simulink model "Parm_track_ieee"  (R2021a)
settings: Solver=ode8  StartTime=0.0  StopTime=FB_current.time(end)  FixedStep=ts  RelTol=1e-3
undefined symbols (not defined in the file): As, Bs, c1, c2, Cs, Ds, k, lambda, LipFT, LipI2T, p, p2, qmax, r1, r2, r3, ts, Tse
libraries: simulink x11
settings Model: SimulationMode=accelerator  Creator=Usuario  LastModifiedBy=pedro
settings SolverCC: AlgebraicLoopSolver=TrustRegion
settings DataIOCC: ExternalInput=FBI(i)  LoadExternalInput=on  SaveOutput=off  SignalLogging=off  DSMLogging=off  SaveTime=off  ReturnWorkspaceOutputs=off
settings DebuggingCC: SFMachineParentedDataDiag=warning  ArithmeticOperatorsInVariantConditions=warning
settings SFSimCC: SimUseLocalCustomCode=off  CustomCodeUndefinedFunction=UseInterfaceOnly
settings RTWCC: RTWUseLocalCustomCode=off

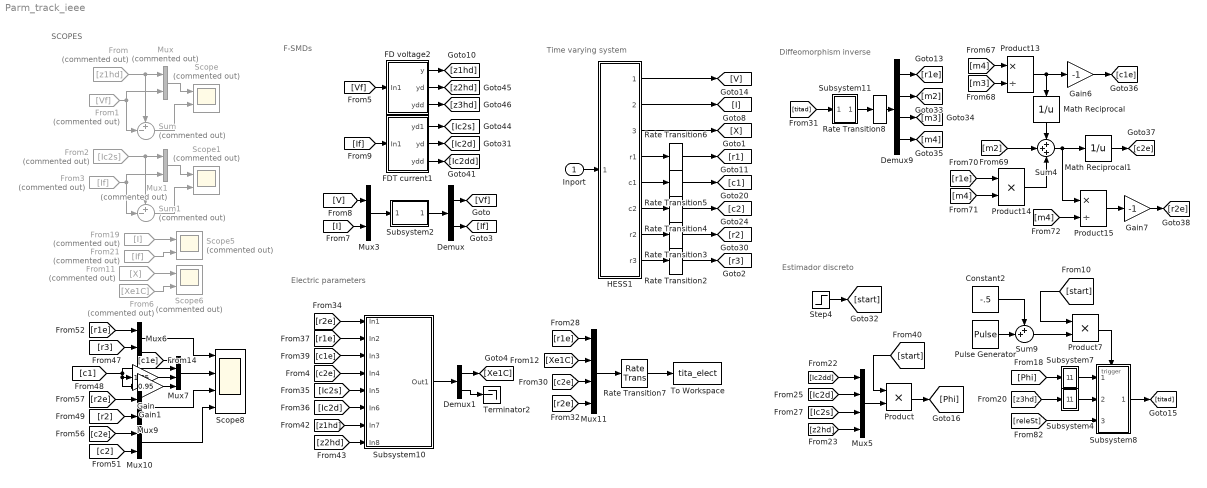
== system Parm_track_ieee ==
  note: Estimador discreto
  note: SCOPES
  note: F-SMDs
  note: Time varying system
  note: Diffeomorphism inverse
  note: Electric parameters
  Inport : Inport
  Constant2 : Constant  Value=-.5
  Demux : Demux  Outputs=2
  Demux1 : Demux  Outputs=2
  Demux9 : Demux
  FD voltage2 : Subsystem
  FDT current1 : Subsystem
  From : From  Commented=on  GotoTag=z1hd
  From1 : From  Commented=on  GotoTag=Vf
  From11 : From  Commented=on  GotoTag=X
  From19 : From  Commented=on  GotoTag=I
  From2 : From  Commented=on  GotoTag=Ic2s
  From21 : From  Commented=on  GotoTag=If
  From3 : From  Commented=on  GotoTag=If
  From6 : From  Commented=on  GotoTag=Xe1C
  Gain : Gain  Gain=1.05
  Gain1 : Gain  Gain=0.95
  Gain6 : Gain  Gain=-1
  Gain7 : Gain  Gain=-1
  HESS1 : Subsystem
  Math Reciprocal : Math  Operator=reciprocal  SignedPower=on  SaturateOnIntegerOverflow=on
  Math Reciprocal1 : Math  Operator=reciprocal  SignedPower=on  SaturateOnIntegerOverflow=on
  Mux : Mux  Commented=on  Inputs=2
  Mux1 : Mux  Commented=on  Inputs=2
  Mux{3,6,9..10} (4 alike) : Mux  Inputs=2
  Mux11 : Mux
  Mux5 : Mux
  Mux7 : Mux
  Product : Product
  Product13 : Product  Inputs=*/
  Product14 : Product
  Product15 : Product  Inputs=*/
  Product7 : Product
  Pulse Generator : DiscretePulseGenerator  PulseType=Time based  Period=Tse  PulseWidth=50
  Rate Transition{2..6,8} (6 alike) : RateTransition  OutPortSampleTime=Tse
  Rate Transition7 : RateTransition  OutPortSampleTime=Tse*2000
  Scope{,1,5..6} (4 alike) : Scope  Commented=on  NumInputPorts=2
  Scope8 : Scope  NumInputPorts=4
  Step4 : Step  Time=30  SampleTime=0
  Subsystem10 : Subsystem
  Subsystem11 : Subsystem
  Subsystem2 : Subsystem
  Subsystem4 : Subsystem
  Subsystem7 : Subsystem
  Subsystem8 : Subsystem
  Sum : Sum  Commented=on  Inputs=+-|
  Sum1 : Sum  Commented=on  Inputs=+-|
  Sum4 : Sum  Inputs=+++
  Sum9 : Sum  Inputs=++|
  Terminator2 : Terminator
  To Workspace : ToWorkspace  VariableName=tita_elect  SaveFormat=Structure With Time  SampleTime=-1
  wires:
  Subsystem2/1(Out1) -> Demux/1
  Demux/1 -> [Vf]
  [V] -> Mux3/1
  Demux/2 -> [If]
  Mux3/1 -> Subsystem2/1(In1)
  HESS1/1(Tensión) -> [V]
  HESS1/2(Corriente) -> [I]
  FD voltage2/2(yd) -> [z2hd]
  FDT current1/1(yd1) -> [Ic2s]
  FD voltage2/1(y) -> [z1hd]
  FDT current1/2(yd) -> [Ic2d]
  [Vf] -> FD voltage2/1(In1)
  FDT current1/3(ydd) -> [Ic2dd]
  [I] -> Mux3/2
  [If] -> FDT current1/1(In1)
  FD voltage2/3(ydd) -> [z3hd]
  Inport/1 -> HESS1/1(Inport)
  HESS1/5(c1) -> Rate Transition5/1
  HESS1/4(r1) -> Rate Transition6/1
  HESS1/6(c2) -> Rate Transition4/1
  HESS1/8(r3) -> Rate Transition2/1
  HESS1/7(r2) -> Rate Transition3/1
  HESS1/3("Estados ") -> [X]
  From/1 -> Mux/1, Sum/1
  From1/1 -> Sum/2, Mux/2
  Mux/1 -> Scope/1
  Sum/1 -> Scope/2
  Sum1/1 -> Scope1/2
  Mux1/1 -> Scope1/1
  From3/1 -> Mux1/2, Sum1/2
  From2/1 -> Sum1/1, Mux1/1
  [releSt] -> Subsystem8/3(In3)
  Subsystem8/1(Output) -> [titad]
  Subsystem4/1(Out1) -> Subsystem8/2(In2)
  Pulse Generator/1 -> Sum9/2
  [Ic2dd] -> Mux5/1
  Mux5/1 -> Product/2
  [z2hd] -> Mux5/4
  Product/1 -> [Phi]
  [z3hd] -> Subsystem4/1(In1)
  Sum9/1 -> Product7/2
  [Ic2s] -> Mux5/3
  Subsystem7/1(Out1) -> Subsystem8/1(In1)
  [Ic2d] -> Mux5/2
  [Phi] -> Subsystem7/1(In1)
  Step4/1 -> [start]
  [m4] -> Product13/1
  [m4] -> Product15/2
  Math Reciprocal/1 -> Sum4/1
  Demux9/3 -> [m3]
  Math Reciprocal1/1 -> [c2e]
  Demux9/1 -> [r1e]
  Demux9/4 -> [m4]
  [m4] -> Product14/2
  [m3] -> Product13/2
  Gain7/1 -> [r2e]
  [r1e] -> Product14/1
  Demux9/2 -> [m2]
  Product15/1 -> Gain7/1
  [m2] -> Sum4/2
  Gain6/1 -> [c1e]
  Mux9/1 -> Scope8/3
  Mux7/1 -> Scope8/2
  Gain/1 -> Mux7/3
  [c2] -> Mux10/2
  [c2e] -> Mux10/1
  [r2e] -> Mux9/1
  [r3] -> Mux6/2
  Gain1/1 -> Mux7/4
  Mux6/1 -> Scope8/1
  [r2] -> Mux9/2
  Mux10/1 -> Scope8/4
  [c1] -> Mux7/2, Gain1/1, Gain/1
  [r1e] -> Mux6/1
  From19/1 -> Scope5/1
  From21/1 -> Scope5/2
  Rate Transition2/1 -> [r3]
  Rate Transition3/1 -> [r2]
  Rate Transition4/1 -> [c2]
  Rate Transition5/1 -> [c1]
  Rate Transition6/1 -> [r1]
  [Xe1C] -> Mux11/2
  [r1e] -> Mux11/1
  [c2e] -> Mux11/3
  [r2e] -> Mux11/4
  Mux11/1 -> Rate Transition7/1
  Rate Transition7/1 -> To Workspace/1
  From11/1 -> Scope6/1
  [c1e] -> Mux7/1
  [titad] -> Subsystem11/1(In1)
  Subsystem11/1(Out1) -> Rate Transition8/1
  Rate Transition8/1 -> Demux9/1
  Product13/1 -> Math Reciprocal/1, Gain6/1
  Product14/1 -> Sum4/3
  Sum4/1 -> Product15/1, Math Reciprocal1/1
  [start] -> Product7/1
  Constant2/1 -> Sum9/1
  [start] -> Product/1
  Product7/1 -> Subsystem8/Trigger
  [z1hd] -> Subsystem10/7(In7)
  Subsystem10/1(Out1) -> Demux1/1
  [Ic2d] -> Subsystem10/6(In6)
  [z2hd] -> Subsystem10/8(In8)
  [Ic2s] -> Subsystem10/5(In5)
  Demux1/2 -> Terminator2/1
  [r1e] -> Subsystem10/2(In2)
  [c2e] -> Subsystem10/4(In4)
  Demux1/1 -> [Xe1C]
  [r2e] -> Subsystem10/1(In1)
  [c1e] -> Subsystem10/3(In3)
  From6/1 -> Scope6/2

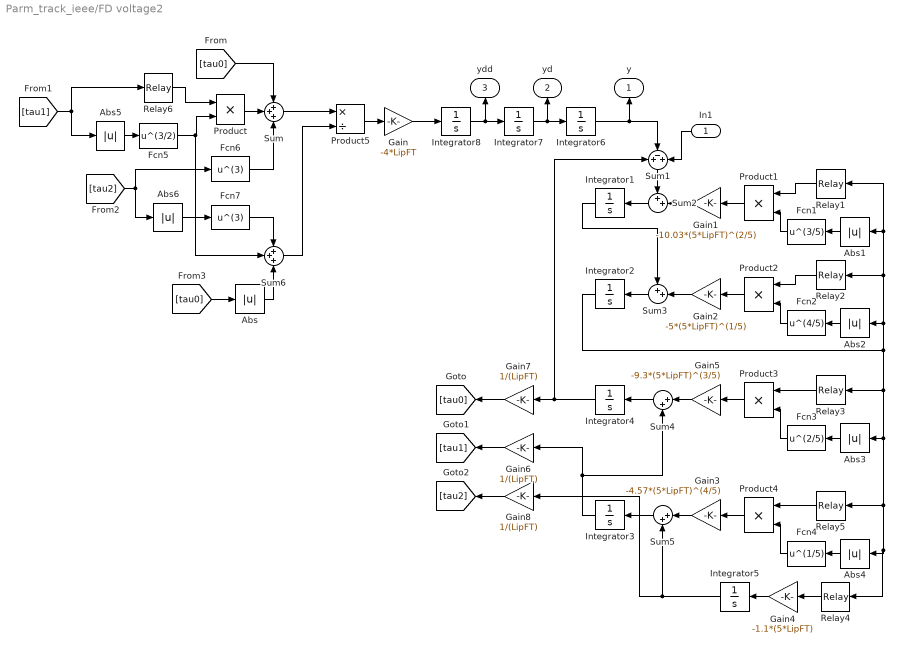
== system Parm_track_ieee/FD voltage2 ==
  In1 : Inport
  Abs{,1..6} (7 alike) : Abs
  Fcn1 : Fcn  Expr=u^(3/5)
  Fcn2 : Fcn  Expr=u^(4/5)
  Fcn3 : Fcn  Expr=u^(2/5)
  Fcn4 : Fcn  Expr=u^(1/5)
  Fcn5 : Fcn  Expr=u^(3/2)
  Fcn6 : Fcn  Expr=u^(3)
  Fcn7 : Fcn  Expr=u^(3)
  Gain : Gain  Gain=-4*LipFT
  Gain1 : Gain  Gain=-10.03*(5*LipFT)^(2/5)
  Gain2 : Gain  Gain=-5*(5*LipFT)^(1/5)
  Gain3 : Gain  Gain=-4.57*(5*LipFT)^(4/5)
  Gain4 : Gain  Gain=-1.1*(5*LipFT)
  Gain5 : Gain  Gain=-9.3*(5*LipFT)^(3/5)
  Gain6 : Gain  Gain=1/(LipFT)
  Gain7 : Gain  Gain=1/(LipFT)
  Gain8 : Gain  Gain=1/(LipFT)
  Integrator{1..3,5,7..8} (6 alike) : Integrator
  Integrator4 : Integrator  InitialCondition=0.001
  Integrator6 : Integrator  InitialCondition=450
  Product{,1..4} (5 alike) : Product
  Product5 : Product  Inputs=*/
  Relay{1..6} (6 alike) : Relay  OnSwitchValue=0  OffSwitchValue=0  OffOutputValue=-1
  Sum : Sum  Inputs=+++
  Sum1 : Sum  Inputs=+-+
  Sum2 : Sum  Inputs=++|
  Sum3 : Sum  Inputs=++|
  Sum4 : Sum  Inputs=|++
  Sum5 : Sum  Inputs=|++
  Sum6 : Sum  Inputs=+++
  y : Outport  VectorParamsAs1DForOutWhenUnconnected=off
  yd : Outport  Port=2  VectorParamsAs1DForOutWhenUnconnected=off
  ydd : Outport  Port=3  VectorParamsAs1DForOutWhenUnconnected=off
  wires:
  In1/1 -> Sum1/3
  Gain1/1 -> Sum2/2
  Sum2/1 -> Integrator1/1
  Sum1/1 -> Sum2/1
  Relay1/1 -> Product1/1
  Product1/1 -> Gain1/1
  Fcn1/1 -> Product1/2
  Abs1/1 -> Fcn1/1
  Sum3/1 -> Integrator2/1
  Abs2/1 -> Fcn2/1
  Fcn2/1 -> Product2/2
  Product2/1 -> Gain2/1
  Relay2/1 -> Product2/1
  Gain2/1 -> Sum3/2
  Integrator1/1 -> Sum3/1
  Integrator2/1 -> Relay1/1, Abs1/1, Relay2/1, Abs2/1, Relay4/1, Abs4/1, Relay5/1, Abs3/1, Relay3/1
  Integrator5/1 -> Gain8/1, Sum5/2
  Abs4/1 -> Fcn4/1
  Relay3/1 -> Product3/1
  Sum5/1 -> Integrator3/1
  Product3/1 -> Gain5/1
  Gain5/1 -> Sum4/1
  Relay4/1 -> Gain4/1
  Gain3/1 -> Sum5/1
  Gain4/1 -> Integrator5/1
  Fcn3/1 -> Product3/2
  Fcn4/1 -> Product4/2
  Integrator3/1 -> Gain6/1, Sum4/2
  Sum4/1 -> Integrator4/1
  Abs3/1 -> Fcn3/1
  Product4/1 -> Gain3/1
  Relay5/1 -> Product4/1
  Integrator4/1 -> Gain7/1, Sum1/1
  Integrator7/1 -> yd/1, Integrator6/1
  Integrator8/1 -> ydd/1, Integrator7/1
  Integrator6/1 -> y/1, Sum1/2
  Gain/1 -> Integrator8/1
  Abs5/1 -> Fcn5/1
  Relay6/1 -> Product/1
  Fcn5/1 -> Sum6/2, Product/2
  [tau1] -> Abs5/1, Relay6/1
  [tau2] -> Fcn6/1, Abs6/1
  Product/1 -> Sum/2
  [tau0] -> Sum/1
  Fcn6/1 -> Sum/3
  Product5/1 -> Gain/1
  Sum/1 -> Product5/1
  Sum6/1 -> Product5/2
  Abs6/1 -> Fcn7/1
  Fcn7/1 -> Sum6/1
  [tau0] -> Abs/1
  Abs/1 -> Sum6/3
  Gain7/1 -> [tau0]
  Gain8/1 -> [tau2]
  Gain6/1 -> [tau1]

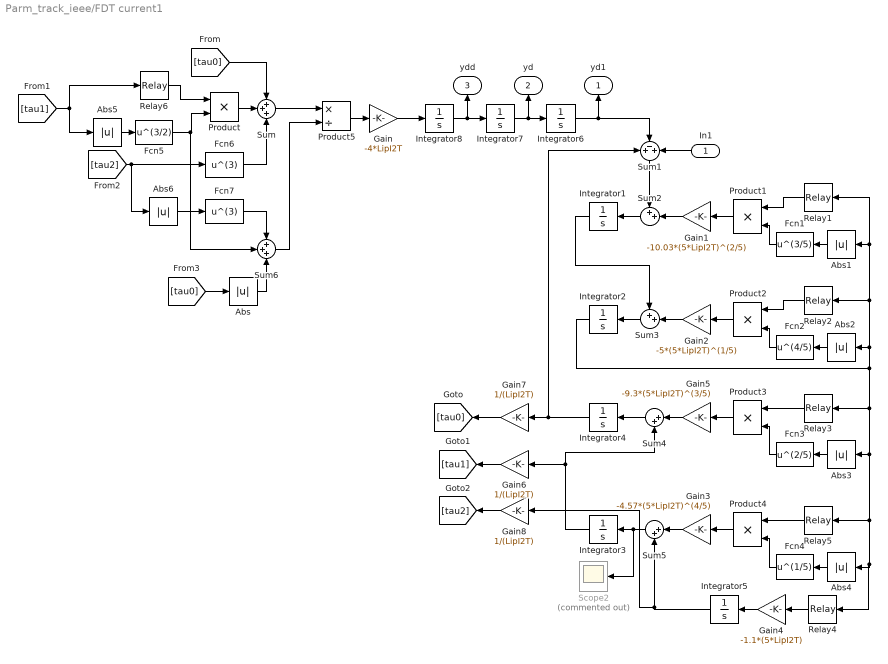
== system Parm_track_ieee/FDT current1 ==
  In1 : Inport
  Abs{,1..6} (7 alike) : Abs
  Fcn1 : Fcn  Expr=u^(3/5)
  Fcn2 : Fcn  Expr=u^(4/5)
  Fcn3 : Fcn  Expr=u^(2/5)
  Fcn4 : Fcn  Expr=u^(1/5)
  Fcn5 : Fcn  Expr=u^(3/2)
  Fcn6 : Fcn  Expr=u^(3)
  Fcn7 : Fcn  Expr=u^(3)
  Gain : Gain  Gain=-4*LipI2T
  Gain1 : Gain  Gain=-10.03*(5*LipI2T)^(2/5)
  Gain2 : Gain  Gain=-5*(5*LipI2T)^(1/5)
  Gain3 : Gain  Gain=-4.57*(5*LipI2T)^(4/5)
  Gain4 : Gain  Gain=-1.1*(5*LipI2T)
  Gain5 : Gain  Gain=-9.3*(5*LipI2T)^(3/5)
  Gain6 : Gain  Gain=1/(LipI2T)
  Gain7 : Gain  Gain=1/(LipI2T)
  Gain8 : Gain  Gain=1/(LipI2T)
  Integrator{1..3,5..8} (7 alike) : Integrator
  Integrator4 : Integrator  InitialCondition=0.001
  Product{,1..4} (5 alike) : Product
  Product5 : Product  Inputs=*/
  Relay{1..6} (6 alike) : Relay  OnSwitchValue=0  OffSwitchValue=0  OffOutputValue=-1
  Scope2 : Scope  Commented=on
  Sum : Sum  Inputs=+++
  Sum1 : Sum  Inputs=+-+
  Sum2 : Sum  Inputs=++|
  Sum3 : Sum  Inputs=++|
  Sum4 : Sum  Inputs=|++
  Sum5 : Sum  Inputs=|++
  Sum6 : Sum  Inputs=+++
  yd1 : Outport  VectorParamsAs1DForOutWhenUnconnected=off
  yd : Outport  Port=2  VectorParamsAs1DForOutWhenUnconnected=off
  ydd : Outport  Port=3  VectorParamsAs1DForOutWhenUnconnected=off
  wires:
  Gain6/1 -> [tau1]
  Gain8/1 -> [tau2]
  Gain7/1 -> [tau0]
  Abs/1 -> Sum6/3
  [tau0] -> Abs/1
  Fcn7/1 -> Sum6/1
  Abs6/1 -> Fcn7/1
  Sum6/1 -> Product5/2
  Sum/1 -> Product5/1
  Product5/1 -> Gain/1
  Fcn6/1 -> Sum/3
  [tau0] -> Sum/1
  Product/1 -> Sum/2
  [tau2] -> Fcn6/1, Abs6/1
  [tau1] -> Relay6/1, Abs5/1
  Fcn5/1 -> Product/2, Sum6/2
  Relay6/1 -> Product/1
  Abs5/1 -> Fcn5/1
  Gain/1 -> Integrator8/1
  Integrator6/1 -> Sum1/2, yd1/1
  Integrator8/1 -> ydd/1, Integrator7/1
  Integrator7/1 -> Integrator6/1, yd/1
  Integrator4/1 -> Sum1/1, Gain7/1
  Relay5/1 -> Product4/1
  Product4/1 -> Gain3/1
  Abs3/1 -> Fcn3/1
  Sum4/1 -> Integrator4/1
  Integrator3/1 -> Gain6/1, Sum4/2
  Fcn4/1 -> Product4/2
  Fcn3/1 -> Product3/2
  Gain4/1 -> Integrator5/1
  Gain3/1 -> Sum5/1
  Relay4/1 -> Gain4/1
  Gain5/1 -> Sum4/1
  Product3/1 -> Gain5/1
  Sum5/1 -> Integrator3/1, Scope2/1
  Relay3/1 -> Product3/1
  Abs4/1 -> Fcn4/1
  Integrator5/1 -> Gain8/1, Sum5/2
  Integrator2/1 -> Abs2/1, Relay2/1, Abs1/1, Relay1/1, Relay3/1, Abs3/1, Relay5/1, Abs4/1, Relay4/1
  Integrator1/1 -> Sum3/1
  Gain2/1 -> Sum3/2
  Relay2/1 -> Product2/1
  Product2/1 -> Gain2/1
  Fcn2/1 -> Product2/2
  Abs2/1 -> Fcn2/1
  Sum3/1 -> Integrator2/1
  Abs1/1 -> Fcn1/1
  Fcn1/1 -> Product1/2
  Product1/1 -> Gain1/1
  Relay1/1 -> Product1/1
  Sum1/1 -> Sum2/1
  Sum2/1 -> Integrator1/1
  Gain1/1 -> Sum2/2
  In1/1 -> Sum1/3

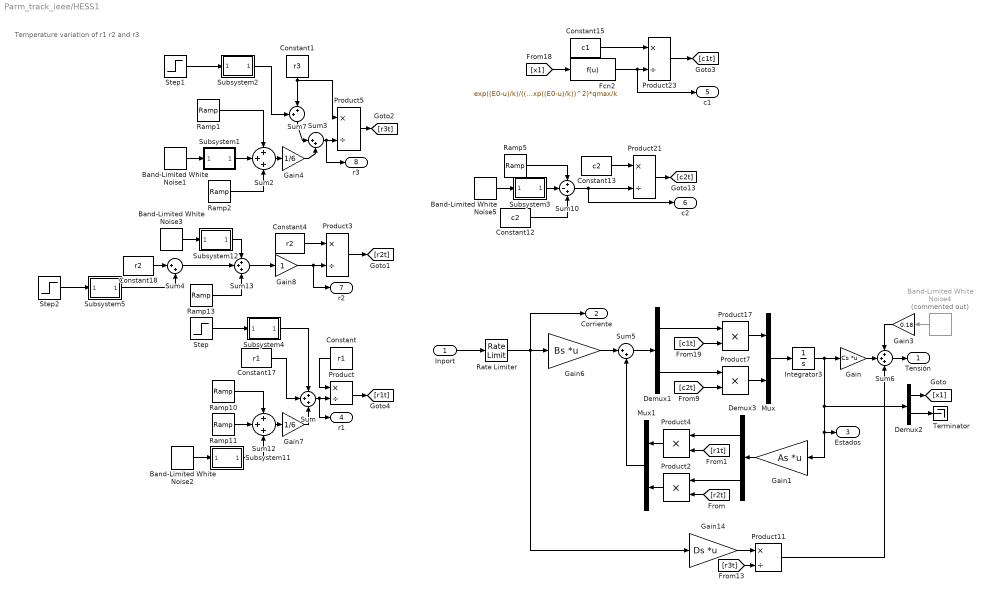
== system Parm_track_ieee/HESS1 ==
  note: Temperature variation of r1 r2 and r3
  Inport : Inport
  Band-Limited White Noise1 : simulink/Sources/Band-Limited White Noise  Cov=[0.35e-8]  Ts=1000*ts  seed=[23341]
  Band-Limited White Noise2 : simulink/Sources/Band-Limited White Noise  Cov=[0.35e-8]  Ts=1000*ts  seed=[23341]
  Band-Limited White Noise3 : simulink/Sources/Band-Limited White Noise  Cov=10  Ts=ts*1000  seed=[23341]
  Band-Limited White Noise4 : simulink/Sources/Band-Limited White Noise  Commented=on  Cov=[1*0.2e-7]  Ts=ts/20  seed=[21741]
  Band-Limited White Noise5 : simulink/Sources/Band-Limited White Noise  Cov=[0.35e-4]  Ts=1000*ts  seed=[23341]
  Constant : Constant  Value=r1
  Constant1 : Constant  Value=r3
  Constant12 : Constant  Value=c2
  Constant13 : Constant  Value=c2
  Constant15 : Constant  Value=c1
  Constant17 : Constant  Value=r1
  Constant18 : Constant  Value=r2
  Constant4 : Constant  Value=r2
  Demux1 : Demux  Outputs=2
  Demux2 : Demux  Outputs=2
  Demux3 : Demux  Outputs=2
  Fcn2 : Fcn  Expr=exp((E0-u)/k)/((1+exp((E0-u)/k))^2)*qmax/k
  Gain : Gain  Gain=Cs  Multiplication=Matrix(K*u) (u vector)
  Gain1 : Gain  Gain=As  Multiplication=Matrix(K*u) (u vector)
  Gain14 : Gain  Gain=Ds  Multiplication=Matrix(K*u) (u vector)
  Gain3 : Gain  Gain=0.18
  Gain4 : Gain  Gain=1/6
  Gain6 : Gain  Gain=Bs  Multiplication=Matrix(K*u)
  Gain7 : Gain  Gain=1/6
  Gain8 : Gain
  Integrator3 : Integrator  InitialCondition=[400 0]%[492 0]%[456.8;0][452 0]
  Mux : Mux  Inputs=2
  Mux1 : Mux  Inputs=2
  Product{,3,5,11,21,23} (6 alike) : Product  Inputs=*/
  Product{2,4,7,17} (4 alike) : Product
  Ramp1 : simulink/Sources/Ramp  slope=(2e-6)/3  start=30  InitialOutput=0
  Ramp10 : simulink/Sources/Ramp  slope=(2e-6)/3  start=30  InitialOutput=0
  Ramp11 : simulink/Sources/Ramp  slope=-0.5e-7%-2e-5  start=600  InitialOutput=0
  Ramp13 : simulink/Sources/Ramp  slope=-(1.883912823894165e-06)/6  start=0  InitialOutput=0
  Ramp2 : simulink/Sources/Ramp  slope=0.5e-8%-2e-5  start=600  InitialOutput=0
  Ramp5 : simulink/Sources/Ramp  slope=0.001  start=200  InitialOutput=0
  Rate Limiter : RateLimiter  RisingSlewLimit=30  FallingSlewLimit=-30  SampleTimeMode=inherited
  Step : Step  Time=0.9e4  After=0%-520  SampleTime=0
  Step1 : Step  Time=2400  After=0%0.1*r3  SampleTime=0
  Step2 : Step  Time=5400  After=0%0.3*r2  SampleTime=0
  Subsystem1 : Subsystem
  Subsystem11 : Subsystem
  Subsystem12 : Subsystem
  Subsystem2 : Subsystem
  Subsystem3 : Subsystem
  Subsystem4 : Subsystem
  Subsystem5 : Subsystem
  Sum{,2,6,12..13} (5 alike) : Sum  Inputs=+++
  Sum10 : Sum  Inputs=+-+
  Sum3 : Sum  Inputs=|++
  Sum4 : Sum  Inputs=|++
  Sum5 : Sum  Inputs=|++
  Sum7 : Sum  Inputs=++|
  Terminator : Terminator
  Tensión : Outport  VectorParamsAs1DForOutWhenUnconnected=off
  Corriente : Outport  Port=2  VectorParamsAs1DForOutWhenUnconnected=off
  "Estados " : Outport  Port=3  VectorParamsAs1DForOutWhenUnconnected=off
  r1 : Outport  Port=4  VectorParamsAs1DForOutWhenUnconnected=off
  c1 : Outport  Port=5  VectorParamsAs1DForOutWhenUnconnected=off
  c2 : Outport  Port=6  VectorParamsAs1DForOutWhenUnconnected=off
  r2 : Outport  Port=7  VectorParamsAs1DForOutWhenUnconnected=off
  r3 : Outport  Port=8  VectorParamsAs1DForOutWhenUnconnected=off
  wires:
  Gain8/1 -> r2/1, Product3/2
  Constant17/1 -> Sum/2
  Gain7/1 -> Sum/3
  Sum12/1 -> Gain7/1
  Sum/1 -> Product/2, r1/1
  Demux2/1 -> [x1]
  Ramp13/1 -> Sum13/3
  Product3/1 -> [r2t]
  Constant4/1 -> Product3/1
  Sum13/1 -> Gain8/1
  Subsystem12/1(Out1) -> Sum13/1
  Product/1 -> [r1t]
  Constant/1 -> Product/1
  Gain6/1 -> Sum5/1
  Gain/1 -> Sum6/2
  Gain3/1 -> Sum6/1
  Band-Limited White Noise4/1 -> Gain3/1
  Fcn2/1 -> c1/1, Product23/2
  Band-Limited White Noise2/1 -> Subsystem11/1(In1)
  Subsystem11/1(Out1) -> Sum12/3
  Ramp11/1 -> Sum12/2
  Ramp10/1 -> Sum12/1
  Product23/1 -> [c1t]
  Constant15/1 -> Product23/1
  Product21/1 -> [c2t]
  Constant13/1 -> Product21/1
  Constant12/1 -> Sum10/3
  Sum10/1 -> Product21/2, c2/1
  Ramp5/1 -> Sum10/1
  Demux1/1 -> Product17/1
  [c1t] -> Product17/2
  Product17/1 -> Mux/1
  [x1] -> Fcn2/1
  [c2t] -> Product7/2
  Product7/1 -> Mux/2
  Inport/1 -> Rate Limiter/1
  [r3t] -> Product11/2
  Gain14/1 -> Product11/1
  [r2t] -> Product2/2
  Gain1/1 -> Demux3/1
  Mux1/1 -> Sum5/2
  Mux/1 -> Integrator3/1
  Demux1/2 -> Product7/1
  Sum5/1 -> Demux1/1
  Sum6/1 -> Tensión/1
  Product11/1 -> Sum6/3
  Integrator3/1 -> Gain1/1, "Estados "/1, Demux2/1, Gain/1
  Demux3/2 -> Product2/1
  Product2/1 -> Mux1/2
  Product4/1 -> Mux1/1
  Demux3/1 -> Product4/1
  [r1t] -> Product4/2
  Sum3/1 -> Product5/2, r3/1
  Product5/1 -> [r3t]
  Ramp1/1 -> Sum2/1
  Ramp2/1 -> Sum2/3
  Subsystem1/1(Out1) -> Sum2/2
  Band-Limited White Noise1/1 -> Subsystem1/1(In1)
  Sum2/1 -> Gain4/1
  Constant1/1 -> Sum7/2, Product5/1
  Gain4/1 -> Sum3/2
  Demux2/2 -> Terminator/1
  Subsystem3/1(Out1) -> Sum10/2
  Band-Limited White Noise5/1 -> Subsystem3/1(In1)
  Band-Limited White Noise3/1 -> Subsystem12/1(In1)
  Step/1 -> Subsystem4/1(In1)
  Sum7/1 -> Sum3/1
  Step1/1 -> Subsystem2/1(In1)
  Subsystem2/1(Out1) -> Sum7/1
  Subsystem4/1(Out1) -> Sum/1
  Constant18/1 -> Sum4/1
  Sum4/1 -> Sum13/2
  Step2/1 -> Subsystem5/1(In1)
  Subsystem5/1(Out1) -> Sum4/2
  Rate Limiter/1 -> Gain14/1, Corriente/1, Gain6/1

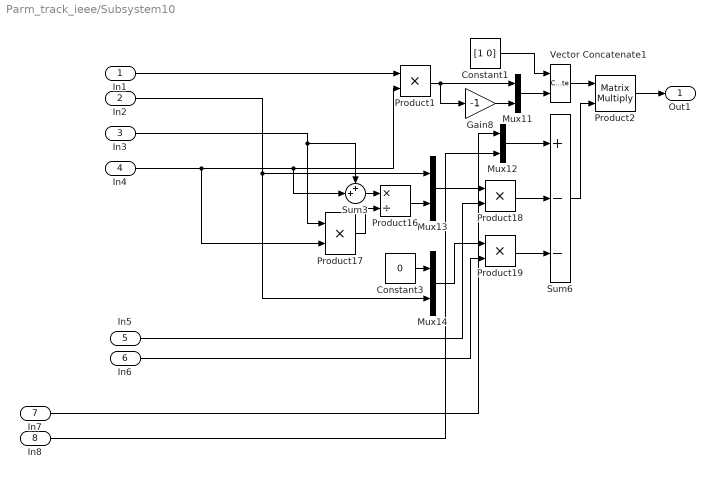
== system Parm_track_ieee/Subsystem10 ==
  In1 : Inport
  In2 : Inport  Port=2
  In3 : Inport  Port=3
  In4 : Inport  Port=4
  In5 : Inport  Port=5
  In6 : Inport  Port=6
  In7 : Inport  Port=7
  In8 : Inport  Port=8
  Constant1 : Constant  Value=[1 0]
  Constant3 : Constant  Value=0
  Gain8 : Gain  Gain=-1
  Mux{11..14} (4 alike) : Mux  Inputs=2
  Product{1,17..19} (4 alike) : Product
  Product16 : Product  Inputs=*/
  Product2 : Product  Multiplication=Matrix(*)
  Sum3 : Sum  Inputs=++|
  Sum6 : Sum  Inputs=+--
  Vector Concatenate1 : Concatenate  Mode=Multidimensional array  ConcatenateDimension=2
  Out1 : Outport
  wires:
  In2/1 -> Mux14/2, Mux13/1
  In3/1 -> Sum3/1, Product17/1
  In7/1 -> Mux12/1
  Mux14/1 -> Product19/1
  Gain8/1 -> Mux11/2
  Mux11/1 -> Vector Concatenate1/2
  Product17/1 -> Product16/2
  Product1/1 -> Mux11/1, Gain8/1
  Product16/1 -> Mux13/2
  Product18/1 -> Sum6/2
  In8/1 -> Mux12/2
  Constant3/1 -> Mux14/1
  Product19/1 -> Sum6/3
  In6/1 -> Product19/2
  Mux13/1 -> Product18/1
  In1/1 -> Product1/1
  Sum6/1 -> Product2/2
  Sum3/1 -> Product16/1
  Product2/1 -> Out1/1
  Mux12/1 -> Sum6/1
  Vector Concatenate1/1 -> Product2/1
  In5/1 -> Product18/2
  In4/1 -> Product17/2, Sum3/2, Product1/2
  Constant1/1 -> Vector Concatenate1/1

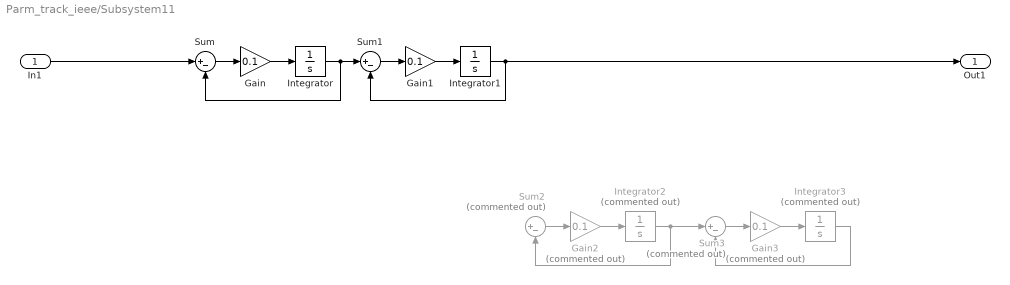
== system Parm_track_ieee/Subsystem11 ==
  In1 : Inport
  Gain : Gain  Gain=0.1
  Gain1 : Gain  Gain=0.1
  Gain2 : Gain  Commented=on  Gain=0.1
  Gain3 : Gain  Commented=on  Gain=0.1
  Integrator : Integrator
  Integrator1 : Integrator
  Integrator2 : Integrator  Commented=on
  Integrator3 : Integrator  Commented=on
  Sum : Sum  Inputs=|+-
  Sum1 : Sum  Inputs=|+-
  Sum2 : Sum  Commented=on  Inputs=|+-
  Sum3 : Sum  Commented=on  Inputs=|+-
  Out1 : Outport
  wires:
  Gain3/1 -> Integrator3/1
  Integrator3/1 -> Sum3/2
  Sum3/1 -> Gain3/1
  Sum2/1 -> Gain2/1
  Integrator2/1 -> Sum2/2, Sum3/1
  Gain2/1 -> Integrator2/1
  Gain1/1 -> Integrator1/1
  Sum1/1 -> Gain1/1
  In1/1 -> Sum/1
  Sum/1 -> Gain/1
  Integrator/1 -> Sum/2, Sum1/1
  Gain/1 -> Integrator/1
  Integrator1/1 -> Out1/1, Sum1/2

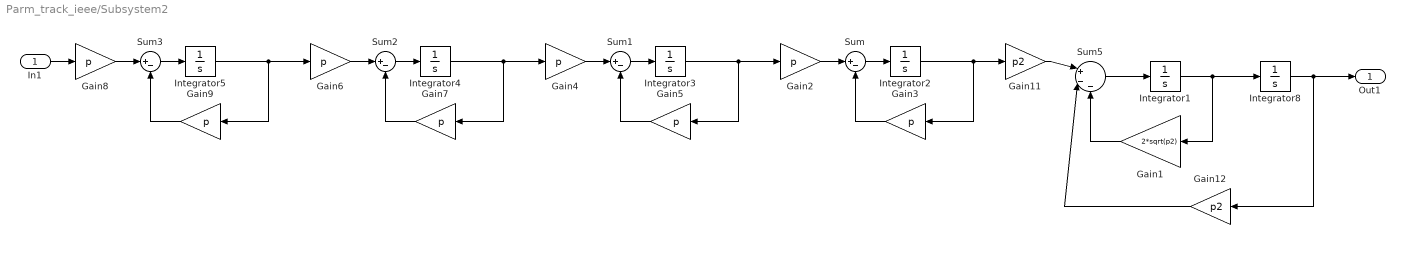
== system Parm_track_ieee/Subsystem2 ==
  In1 : Inport
  Gain1 : Gain  Gain=2*sqrt(p2)
  Gain11 : Gain  Gain=p2
  Gain12 : Gain  Gain=p2
  Gain{2..9} (8 alike) : Gain  Gain=p
  Integrator1 : Integrator  InitialCondition=[0 0 ]
  Integrator{2..5} (4 alike) : Integrator  InitialCondition=[450 0]
  Integrator8 : Integrator  InitialCondition=[450 0 ]
  Sum{,1..3} (4 alike) : Sum  Inputs=|+-
  Sum5 : Sum  Inputs=|+--
  Out1 : Outport  VectorParamsAs1DForOutWhenUnconnected=off
  wires:
  Integrator8/1 -> Gain12/1, Out1/1
  Gain11/1 -> Sum5/1
  Gain12/1 -> Sum5/2
  Sum5/1 -> Integrator1/1
  Integrator1/1 -> Gain1/1, Integrator8/1
  Gain1/1 -> Sum5/3
  Integrator2/1 -> Gain3/1, Gain11/1
  Gain2/1 -> Sum/1
  Sum/1 -> Integrator2/1
  Gain3/1 -> Sum/2
  Gain5/1 -> Sum1/2
  Sum1/1 -> Integrator3/1
  Gain4/1 -> Sum1/1
  Integrator3/1 -> Gain2/1, Gain5/1
  Integrator4/1 -> Gain4/1, Gain7/1
  Gain6/1 -> Sum2/1
  Sum2/1 -> Integrator4/1
  Gain7/1 -> Sum2/2
  Gain9/1 -> Sum3/2
  Sum3/1 -> Integrator5/1
  Gain8/1 -> Sum3/1
  Integrator5/1 -> Gain6/1, Gain9/1
  In1/1 -> Gain8/1

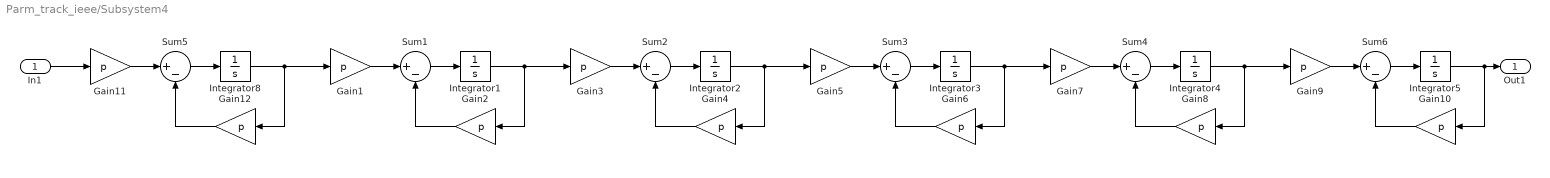
== system Parm_track_ieee/Subsystem4 ==
  In1 : Inport
  Gain{1..12} (12 alike) : Gain  Gain=p
  Integrator{1..5,8} (6 alike) : Integrator
  Sum{1..6} (6 alike) : Sum  Inputs=|+-
  Out1 : Outport  VectorParamsAs1DForOutWhenUnconnected=off
  wires:
  Integrator1/1 -> Gain2/1, Gain3/1
  Gain3/1 -> Sum2/1
  Gain4/1 -> Sum2/2
  Sum2/1 -> Integrator2/1
  Sum1/1 -> Integrator1/1
  Gain2/1 -> Sum1/2
  Gain1/1 -> Sum1/1
  Integrator8/1 -> Gain12/1, Gain1/1
  In1/1 -> Gain11/1
  Gain11/1 -> Sum5/1
  Gain12/1 -> Sum5/2
  Sum5/1 -> Integrator8/1
  Sum3/1 -> Integrator3/1
  Gain6/1 -> Sum3/2
  Gain5/1 -> Sum3/1
  Integrator2/1 -> Gain5/1, Gain4/1
  Integrator3/1 -> Gain7/1, Gain6/1
  Gain7/1 -> Sum4/1
  Gain8/1 -> Sum4/2
  Sum4/1 -> Integrator4/1
  Sum6/1 -> Integrator5/1
  Integrator5/1 -> Out1/1, Gain10/1
  Gain10/1 -> Sum6/2
  Gain9/1 -> Sum6/1
  Integrator4/1 -> Gain9/1, Gain8/1

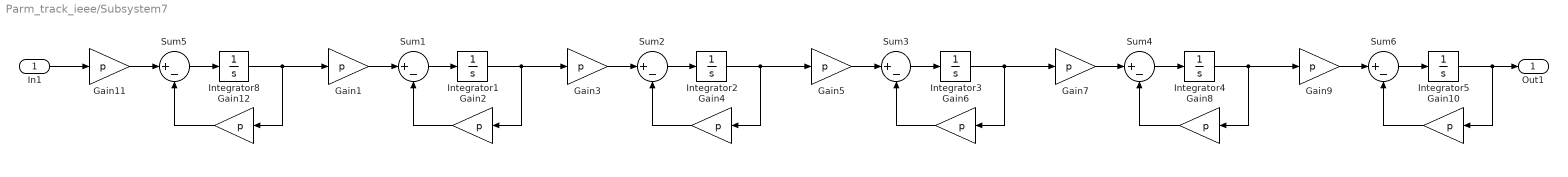
== system Parm_track_ieee/Subsystem7 ==
  In1 : Inport
  Gain{1..12} (12 alike) : Gain  Gain=p
  Integrator{1..5,8} (6 alike) : Integrator
  Sum{1..6} (6 alike) : Sum  Inputs=|+-
  Out1 : Outport  VectorParamsAs1DForOutWhenUnconnected=off
  wires:
  Sum5/1 -> Integrator8/1
  Gain12/1 -> Sum5/2
  Gain11/1 -> Sum5/1
  In1/1 -> Gain11/1
  Integrator8/1 -> Gain1/1, Gain12/1
  Gain1/1 -> Sum1/1
  Gain2/1 -> Sum1/2
  Sum1/1 -> Integrator1/1
  Sum2/1 -> Integrator2/1
  Gain4/1 -> Sum2/2
  Gain3/1 -> Sum2/1
  Integrator1/1 -> Gain3/1, Gain2/1
  Integrator2/1 -> Gain5/1, Gain4/1
  Gain5/1 -> Sum3/1
  Gain6/1 -> Sum3/2
  Sum3/1 -> Integrator3/1
  Sum4/1 -> Integrator4/1
  Gain8/1 -> Sum4/2
  Gain7/1 -> Sum4/1
  Integrator3/1 -> Gain7/1, Gain6/1
  Integrator4/1 -> Gain9/1, Gain8/1
  Gain9/1 -> Sum6/1
  Gain10/1 -> Sum6/2
  Integrator5/1 -> Gain10/1, Out1/1
  Sum6/1 -> Integrator5/1

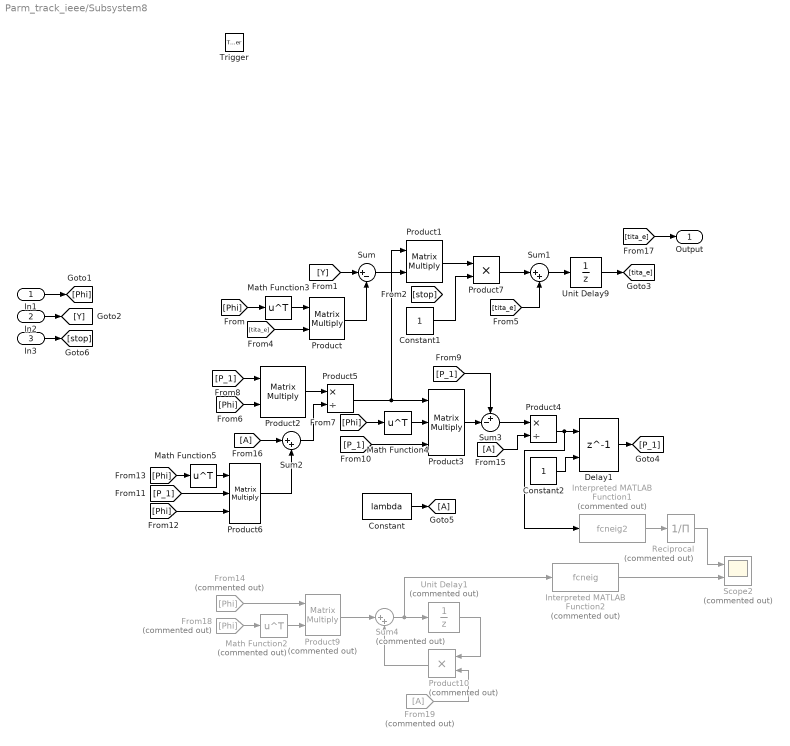
== system Parm_track_ieee/Subsystem8 ==
  In1 : Inport
  In2 : Inport  Port=2
  In3 : Inport  Port=3
  Trigger : TriggerPort  VariantControl=Variant  PortDimensions=1
  Constant : Constant  Value=lambda
  Constant1 : Constant
  Constant2 : Constant
  Delay1 : Delay  DelayLength=1  InitialCondition=eye(4)  ExternalReset=Falling
      settings: InputPortMap=u0,r5
  From14 : From  Commented=on  GotoTag=Phi
  From18 : From  Commented=on  GotoTag=Phi
  From19 : From  Commented=on
  Interpreted MATLAB Function1 : MATLABFcn  Commented=on  MATLABFcn=fcneig2
  Interpreted MATLAB Function2 : MATLABFcn  Commented=on  MATLABFcn=fcneig
  Math Function2 : Math  Commented=on  Operator=transpose  SignedPower=on  SaturateOnIntegerOverflow=on
  Math Function3 : Math  Operator=transpose  SignedPower=on  SaturateOnIntegerOverflow=on
  Math Function4 : Math  Operator=transpose  SignedPower=on  SaturateOnIntegerOverflow=on
  Math Function5 : Math  Operator=transpose  SignedPower=on  SaturateOnIntegerOverflow=on
  Product : Product  Multiplication=Matrix(*)
  Product1 : Product  Multiplication=Matrix(*)
  Product10 : Product  Commented=on
  Product2 : Product  Multiplication=Matrix(*)
  Product3 : Product  Inputs=3  Multiplication=Matrix(*)
  Product4 : Product  Inputs=*/
  Product5 : Product  Inputs=*/
  Product6 : Product  Inputs=3  Multiplication=Matrix(*)
  Product7 : Product
  Product9 : Product  Commented=on  Multiplication=Matrix(*)
  Reciprocal : Product  Commented=on  Inputs=/
  Scope2 : Scope  Commented=on  NumInputPorts=2
  Sum : Sum  Inputs=|+-
  Sum1 : Sum  Inputs=|++
  Sum2 : Sum  Inputs=|++
  Sum3 : Sum  Inputs=+-|
  Sum4 : Sum  Commented=on  Inputs=|++
  Unit Delay1 : UnitDelay  Commented=on  InitialCondition=0*eye(4)  SampleTime=-1  HasFrameUpgradeWarning=on
  Unit Delay9 : UnitDelay  InitialCondition=[0.03;0.006;0.00005;-0.04]  SampleTime=-1  HasFrameUpgradeWarning=on
  Output : Outport
  wires:
  Product1/1 -> Product7/1
  [tita_e] -> Output/1
  [A] -> Product4/2
  Constant/1 -> [A]
  Product4/1 -> Interpreted MATLAB Function1/1, Delay1/1
  [Phi] -> Product2/2
  [Phi] -> Math Function5/1
  Math Function5/1 -> Product6/1
  [Phi] -> Product6/3
  [P_1] -> Product6/2
  Product6/1 -> Sum2/2
  Sum2/1 -> Product5/2
  [A] -> Sum2/1
  Product3/1 -> Sum3/2
  [P_1] -> Product3/3
  Product5/1 -> Product1/1, Product3/1
  Product2/1 -> Product5/1
  [P_1] -> Product2/1
  Math Function4/1 -> Product3/2
  [Phi] -> Math Function4/1
  Delay1/1 -> [P_1]
  Sum3/1 -> Product4/1
  [P_1] -> Sum3/1
  [tita_e] -> Sum1/2
  Sum1/1 -> Unit Delay9/1
  Sum/1 -> Product1/2
  Product/1 -> Sum/2
  [Y] -> Sum/1
  [tita_e] -> Product/2
  Unit Delay9/1 -> [tita_e]
  Math Function3/1 -> Product/1
  [Phi] -> Math Function3/1
  In2/1 -> [Y]
  In1/1 -> [Phi]
  In3/1 -> [stop]
  Product7/1 -> Sum1/1
  Constant1/1 -> Product7/2
  Constant2/1 -> Delay1/2
  From14/1 -> Product9/1
  From18/1 -> Math Function2/1
  Math Function2/1 -> Product9/2
  Product9/1 -> Sum4/1
  Sum4/1 -> Interpreted MATLAB Function2/1, Unit Delay1/1
  Unit Delay1/1 -> Product10/1
  Product10/1 -> Sum4/2
  From19/1 -> Product10/2
  Interpreted MATLAB Function1/1 -> Reciprocal/1
  Reciprocal/1 -> Scope2/1
  Interpreted MATLAB Function2/1 -> Scope2/2

== system Parm_track_ieee/HESS1/Subsystem1 ==
  In1 : Inport
  Gain1 : Gain  Gain=1e-5
  Gain11 : Gain  Gain=1e-5
  Gain12 : Gain  Gain=2*sqrt(1e-5)
  Gain2 : Gain  Gain=400
  Integrator1 : Integrator
  Integrator2 : Integrator
  Integrator8 : Integrator
  Sum1 : Sum  Inputs=|+-
  Sum5 : Sum  Inputs=|+--
  Out1 : Outport  VectorParamsAs1DForOutWhenUnconnected=off
  wires:
  Integrator1/1 -> Gain1/1, Gain2/1
  Integrator8/1 -> Gain12/1, Integrator1/1
  Gain1/1 -> Sum5/2
  Gain11/1 -> Sum5/1
  Gain12/1 -> Sum5/3
  Sum5/1 -> Integrator8/1
  Gain2/1 -> Out1/1
  Integrator2/1 -> Sum1/2, Gain11/1
  In1/1 -> Sum1/1
  Sum1/1 -> Integrator2/1

== system Parm_track_ieee/HESS1/Subsystem11 ==
  In1 : Inport
  Gain1 : Gain  Gain=1e-5
  Gain11 : Gain  Gain=1e-5
  Gain12 : Gain  Gain=2*sqrt(1e-5)
  Gain2 : Gain  Gain=800/3
  Integrator1 : Integrator
  Integrator2 : Integrator
  Integrator8 : Integrator
  Sum1 : Sum  Inputs=|+-
  Sum5 : Sum  Inputs=|+--
  Out1 : Outport  VectorParamsAs1DForOutWhenUnconnected=off
  wires:
  Gain2/1 -> Out1/1
  Sum5/1 -> Integrator8/1
  Gain12/1 -> Sum5/3
  Gain11/1 -> Sum5/1
  In1/1 -> Sum1/1
  Gain1/1 -> Sum5/2
  Integrator8/1 -> Integrator1/1, Gain12/1
  Integrator1/1 -> Gain2/1, Gain1/1
  Integrator2/1 -> Sum1/2, Gain11/1
  Sum1/1 -> Integrator2/1

== system Parm_track_ieee/HESS1/Subsystem12 ==
  In1 : Inport
  Gain1 : Gain  Gain=1e-8
  Gain11 : Gain  Gain=1e-8
  Gain12 : Gain  Gain=2*sqrt(1e-8)
  Gain2 : Gain  Gain=-1
  Integrator : Integrator
  Integrator1 : Integrator
  Integrator8 : Integrator
  Sum : Sum  Inputs=|+-
  Sum5 : Sum  Inputs=|+--
  Out1 : Outport  VectorParamsAs1DForOutWhenUnconnected=off
  wires:
  Sum5/1 -> Integrator8/1
  Gain12/1 -> Sum5/3
  Gain11/1 -> Sum5/1
  Gain1/1 -> Sum5/2
  Integrator8/1 -> Integrator1/1, Gain12/1
  Integrator1/1 -> Gain2/1, Gain1/1
  Gain2/1 -> Out1/1
  Integrator/1 -> Sum/2, Gain11/1
  Sum/1 -> Integrator/1
  In1/1 -> Sum/1

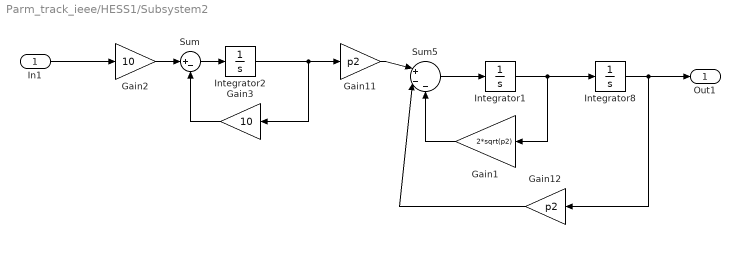
== system Parm_track_ieee/HESS1/Subsystem2 ==
  In1 : Inport
  Gain1 : Gain  Gain=2*sqrt(p2)
  Gain11 : Gain  Gain=p2
  Gain12 : Gain  Gain=p2
  Gain2 : Gain  Gain=10
  Gain3 : Gain  Gain=10
  Integrator1 : Integrator
  Integrator2 : Integrator
  Integrator8 : Integrator
  Sum : Sum  Inputs=|+-
  Sum5 : Sum  Inputs=|+--
  Out1 : Outport  VectorParamsAs1DForOutWhenUnconnected=off
  wires:
  Integrator8/1 -> Gain12/1, Out1/1
  In1/1 -> Gain2/1
  Gain11/1 -> Sum5/1
  Gain12/1 -> Sum5/2
  Sum5/1 -> Integrator1/1
  Integrator1/1 -> Gain1/1, Integrator8/1
  Gain1/1 -> Sum5/3
  Integrator2/1 -> Gain3/1, Gain11/1
  Gain2/1 -> Sum/1
  Sum/1 -> Integrator2/1
  Gain3/1 -> Sum/2

== system Parm_track_ieee/HESS1/Subsystem3 ==
  In1 : Inport
  Gain1 : Gain  Gain=1e-7
  Gain11 : Gain  Gain=1e-7
  Gain12 : Gain  Gain=2*sqrt(1e-7)
  Gain2 : Gain  Gain=250000
  Integrator1 : Integrator
  Integrator2 : Integrator
  Integrator8 : Integrator
  Sum1 : Sum  Inputs=|+-
  Sum5 : Sum  Inputs=|+--
  Out1 : Outport  VectorParamsAs1DForOutWhenUnconnected=off
  wires:
  Sum1/1 -> Integrator2/1
  Integrator2/1 -> Gain11/1, Sum1/2
  Integrator1/1 -> Gain1/1, Gain2/1
  Integrator8/1 -> Gain12/1, Integrator1/1
  Gain1/1 -> Sum5/2
  In1/1 -> Sum1/1
  Gain11/1 -> Sum5/1
  Gain12/1 -> Sum5/3
  Sum5/1 -> Integrator8/1
  Gain2/1 -> Out1/1

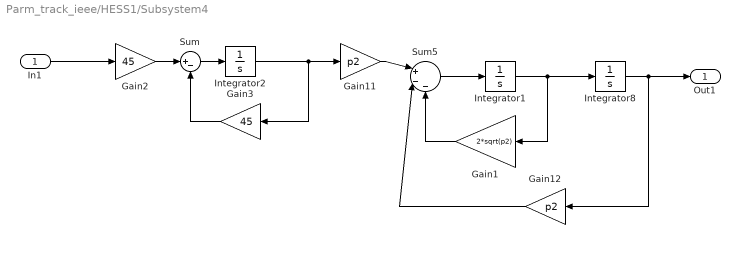
== system Parm_track_ieee/HESS1/Subsystem4 ==
  In1 : Inport
  Gain1 : Gain  Gain=2*sqrt(p2)
  Gain11 : Gain  Gain=p2
  Gain12 : Gain  Gain=p2
  Gain2 : Gain  Gain=45
  Gain3 : Gain  Gain=45
  Integrator1 : Integrator
  Integrator2 : Integrator
  Integrator8 : Integrator
  Sum : Sum  Inputs=|+-
  Sum5 : Sum  Inputs=|+--
  Out1 : Outport  VectorParamsAs1DForOutWhenUnconnected=off
  wires:
  Gain3/1 -> Sum/2
  Sum/1 -> Integrator2/1
  Gain2/1 -> Sum/1
  Integrator2/1 -> Gain11/1, Gain3/1
  Gain1/1 -> Sum5/3
  Integrator1/1 -> Integrator8/1, Gain1/1
  Sum5/1 -> Integrator1/1
  Gain12/1 -> Sum5/2
  Gain11/1 -> Sum5/1
  In1/1 -> Gain2/1
  Integrator8/1 -> Out1/1, Gain12/1

== system Parm_track_ieee/HESS1/Subsystem5 ==
  In1 : Inport
  Gain1 : Gain  Gain=2*sqrt(p2)
  Gain11 : Gain  Gain=p2
  Gain12 : Gain  Gain=p2
  Gain2 : Gain  Gain=45
  Gain3 : Gain  Gain=45
  Integrator1 : Integrator
  Integrator2 : Integrator
  Integrator8 : Integrator
  Sum : Sum  Inputs=|+-
  Sum5 : Sum  Inputs=|+--
  Out1 : Outport  VectorParamsAs1DForOutWhenUnconnected=off
  wires:
  Gain3/1 -> Sum/2
  Sum/1 -> Integrator2/1
  Gain2/1 -> Sum/1
  Integrator2/1 -> Gain11/1, Gain3/1
  Gain1/1 -> Sum5/3
  Integrator1/1 -> Integrator8/1, Gain1/1
  Sum5/1 -> Integrator1/1
  Gain12/1 -> Sum5/2
  Gain11/1 -> Sum5/1
  In1/1 -> Gain2/1
  Integrator8/1 -> Out1/1, Gain12/1
